simulink model "COMP_TIP_LOAD_SYS"  (R2026b)
settings: Solver=VariableStepAuto
undefined symbols (not defined in the file): F_applied
libraries: nesl_utility x1
settings Model: Creator=bhorton  LastModifiedBy=bhorton

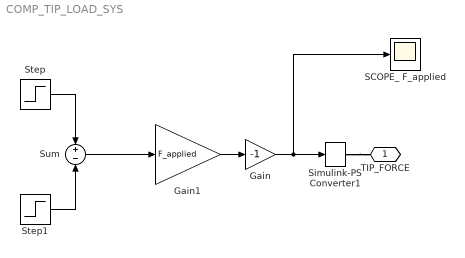
== system COMP_TIP_LOAD_SYS ==
  Gain : Gain  Gain=-1
  Gain1 : Gain  Gain=F_applied
  SCOPE_ F_applied : Scope
  Simulink-PS Converter1 : nesl_utility/Simulink-PS Converter  PhysicalDomain=network_engine_domain  SubClassName=ps_input  LeftPortType=input  RightPortType=output  PseudoPeriodic=off  Frequencies=[]  NoiseDistribution=none  NoiseParameters=[]  Unit=N  AffineConversion=off  FilteringAndDerivatives=provide  SimscapeFilterOrder=2  InputFilterTimeConstant=0.001  UdotUserProvided=0
  Step : Step  Time=3  SampleTime=0
      settings: AttributesFormatString=step @ t = %<Time> (secs)
  Step1 : Step  Time=6  SampleTime=0
      settings: AttributesFormatString=step @ t = %<Time> (secs)
  Sum : Sum  Inputs=+|-
  TIP_FORCE : PMIOPort  Side=Right
  wires:
  Gain/1 -> SCOPE_ F_applied/1, Simulink-PS Converter1/1
  Sum/1 -> Gain1/1
  Step/1 -> Sum/1
  Gain1/1 -> Gain/1
  Step1/1 -> Sum/2
  connections:
  Simulink-PS Converter1/RConn1 -- TIP_FORCE/RConn1
